simulink model "testPEConvSubmodule"  (R2023a)
settings: Solver=VariableStepAuto  StartTime=0.0  StopTime=simu.sim_time  MaxStep=simu.max_stepSize  RelTol=1e-3
values from neighbouring files (symbols this model uses):
  dev = peDevClass("default_mosfet")    [peModelingTest.m]
  i_rms = 25    [peModelingTest.m]
  ma = 0.98    [peModelingTest.m]
libraries: fl_lib x17, nesl_utility x5, simulink x1
settings Model: Creator=smbar  LastModifiedBy=bartonsa
settings DataIOCC: ReturnWorkspaceOutputs=off

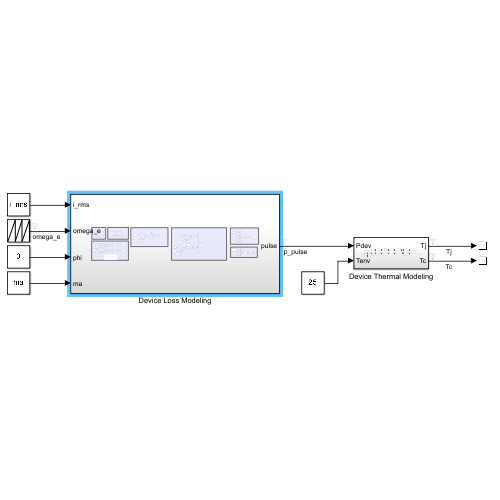
[thumbnail: Simulink's stored preview of the top-level diagram]
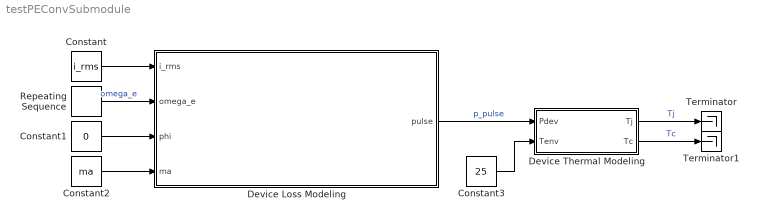
== system testPEConvSubmodule ==
  Constant : Constant  Value=i_rms
  Constant1 : Constant  Value=0
  Constant2 : Constant  Value=ma
  Constant3 : Constant  Value=25
  Device Loss Modeling : Subsystem
  Device Thermal Modeling : Subsystem
  Repeating Sequence : simulink/Sources/Repeating Sequence  rep_seq_t=time_vec  rep_seq_y=omega_e
  Terminator : Terminator
  Terminator1 : Terminator
  wires:
  Constant/1 -> Device Loss Modeling/1(i_rms)
  Repeating Sequence/1 -> Device Loss Modeling/2(omega_e)  "omega_e"
  Constant1/1 -> Device Loss Modeling/3(phi)
  Device Loss Modeling/1(pulse) -> Device Thermal Modeling/1(Pdev)  "p_pulse"
  Constant2/1 -> Device Loss Modeling/4(ma)
  Constant3/1 -> Device Thermal Modeling/2(Tenv)
  Device Thermal Modeling/2(Tc) -> Terminator1/1  "Tc"
  Device Thermal Modeling/1(Tj) -> Terminator/1  "Tj"

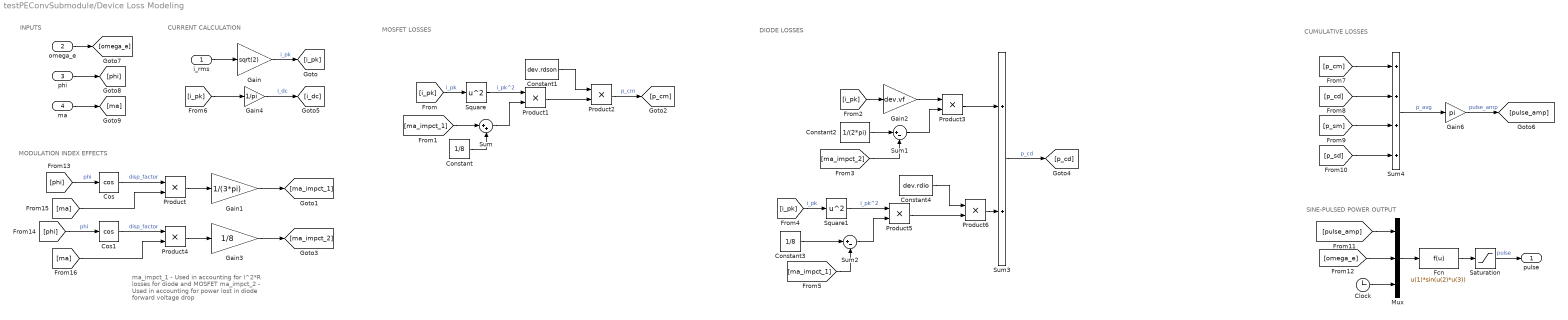
== system testPEConvSubmodule/Device Loss Modeling ==
  note: CUMULATIVE LOSSES
  note: DIODE LOSSES
  note: MOSFET LOSSES
  note: ma_impct_1 - Used in accounting for I^2*R losses for diode and MOSFET
      |
      | ma_impct_2 - Used in accounting for power lost in diode forward voltage drop
  note: MODULATION INDEX EFFECTS
  note: SINE-PULSED POWER OUTPUT
  note: CURRENT CALCULATION
  note: INPUTS
  i_rms : Inport
  omega_e : Inport  Port=2
  phi : Inport  Port=3
  ma : Inport  Port=4
  Clock : Clock
  Constant : Constant  Value=1/8
  Constant1 : Constant  Value=dev.rdson
  Constant2 : Constant  Value=1/(2*pi)
  Constant3 : Constant  Value=1/8
  Constant4 : Constant  Value=dev.rdio
  Cos : Trigonometry  Operator=cos
  Cos1 : Trigonometry  Operator=cos
  Fcn : Fcn  Expr=u(1)*sin(u(2)*u(3))
  Gain : Gain  Gain=sqrt(2)
  Gain1 : Gain  Gain=1/(3*pi)
  Gain2 : Gain  Gain=dev.vf
  Gain3 : Gain  Gain=1/8
  Gain4 : Gain  Gain=1/pi
  Gain6 : Gain  Gain=pi
  Mux : Mux  Inputs=3
  Product{,1..6} (7 alike) : Product
  Saturation : Saturate  UpperLimit=inf  LowerLimit=0
  Square : Math  Operator=square
  Square1 : Math  Operator=square
  Sum : Sum  Inputs=|++
  Sum1 : Sum  Inputs=|+-
  Sum2 : Sum  Inputs=|+-
  Sum3 : Sum
  Sum4 : Sum  Inputs=++++
  pulse : Outport
  wires:
  Product/1 -> Gain1/1
  Sum/1 -> Product1/2
  [pulse_amp] -> Mux/1
  [p_sm] -> Sum4/3
  Gain1/1 -> [ma_impct_1]
  [i_pk] -> Square/1  "i_pk"
  Gain6/1 -> [pulse_amp]  "pulse_amp"
  Sum3/1 -> [p_cd]  "p_cd"
  Product1/1 -> Product2/2
  Cos/1 -> Product/1  "disp_factor"
  Product5/1 -> Product6/2
  [i_pk] -> Square1/1  "i_pk"
  Gain/1 -> [i_pk]  "i_pk"
  Constant/1 -> Sum/2
  Square/1 -> Product1/1  "i_pk^2"
  [ma_impct_2] -> Sum1/2
  i_rms/1 -> Gain/1
  Sum1/1 -> Product3/2
  Product4/1 -> Gain3/1
  Product2/1 -> [p_cm]  "p_cm"
  [i_pk] -> Gain4/1
  Product3/1 -> Sum3/1
  [omega_e] -> Mux/2
  Constant1/1 -> Product2/1
  [i_pk] -> Gain2/1
  Constant4/1 -> Product6/1
  Gain4/1 -> [i_dc]  "i_dc"
  [phi] -> Cos1/1  "phi"
  [p_cd] -> Sum4/2
  [p_cm] -> Sum4/1
  Product6/1 -> Sum3/2
  [p_sd] -> Sum4/4
  [ma] -> Product4/2
  Sum4/1 -> Gain6/1  "p_avg"
  Fcn/1 -> Saturation/1
  [ma_impct_1] -> Sum/1
  Mux/1 -> Fcn/1
  [ma] -> Product/2
  Gain3/1 -> [ma_impct_2]
  Cos1/1 -> Product4/1  "disp_factor"
  Gain2/1 -> Product3/1
  Constant2/1 -> Sum1/1
  Square1/1 -> Product5/1  "i_pk^2"
  Clock/1 -> Mux/3
  Constant3/1 -> Sum2/1
  [ma_impct_1] -> Sum2/2
  Sum2/1 -> Product5/2
  [phi] -> Cos/1  "phi"
  omega_e/1 -> [omega_e]
  Saturation/1 -> pulse/1  "pulse"
  phi/1 -> [phi]
  ma/1 -> [ma]

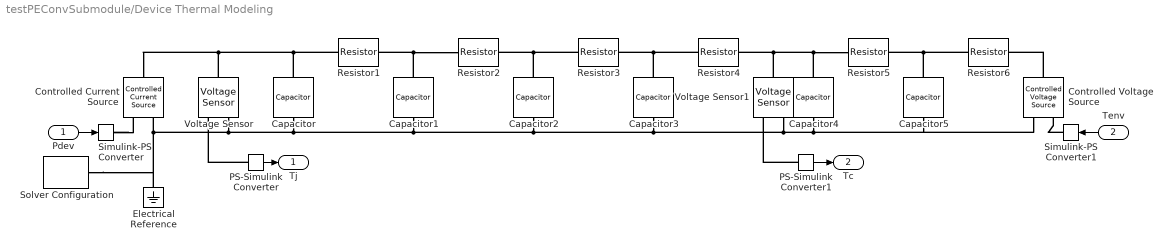
== system testPEConvSubmodule/Device Thermal Modeling ==
  Pdev : Inport
  Tenv : Inport  Port=2
  Capacitor : fl_lib/Electrical/Electrical Elements/Capacitor  c=dev.c(1) F  r=0 Ohm  g=0 1/Ohm  i_specify=off  i_priority=None  i=0 A  i_nominal_specify=off  i_nominal_unit=A  i_nominal_value=1  v_specify=off  v_priority=None  v=0 V  v_nominal_specify=off  v_nominal_unit=V  v_nominal_value=1  vc_specify=off  vc_priority=High  vc=0 V  vc_nominal_specify=off  vc_nominal_unit=V  vc_nominal_value=1
  Capacitor1 : fl_lib/Electrical/Electrical Elements/Capacitor  c=dev.c(2) F  r=0 Ohm  g=0 1/Ohm  i_specify=off  i_priority=None  i=0 A  i_nominal_specify=off  i_nominal_unit=A  i_nominal_value=1  v_specify=off  v_priority=None  v=0 V  v_nominal_specify=off  v_nominal_unit=V  v_nominal_value=1  vc_specify=off  vc_priority=High  vc=0 V  vc_nominal_specify=off  vc_nominal_unit=V  vc_nominal_value=1
  Capacitor2 : fl_lib/Electrical/Electrical Elements/Capacitor  c=dev.c(3) F  r=0 Ohm  g=0 1/Ohm  i_specify=off  i_priority=None  i=0 A  i_nominal_specify=off  i_nominal_unit=A  i_nominal_value=1  v_specify=off  v_priority=None  v=0 V  v_nominal_specify=off  v_nominal_unit=V  v_nominal_value=1  vc_specify=off  vc_priority=High  vc=0 V  vc_nominal_specify=off  vc_nominal_unit=V  vc_nominal_value=1
  Capacitor3 : fl_lib/Electrical/Electrical Elements/Capacitor  c=dev.c(4) F  r=0 Ohm  g=0 1/Ohm  i_specify=off  i_priority=None  i=0 A  i_nominal_specify=off  i_nominal_unit=A  i_nominal_value=1  v_specify=off  v_priority=None  v=0 V  v_nominal_specify=off  v_nominal_unit=V  v_nominal_value=1  vc_specify=off  vc_priority=High  vc=0 V  vc_nominal_specify=off  vc_nominal_unit=V  vc_nominal_value=1
  Capacitor4 : fl_lib/Electrical/Electrical Elements/Capacitor  c=dev.c(5) F  r=0 Ohm  g=0 1/Ohm  i_specify=off  i_priority=None  i=0 A  i_nominal_specify=off  i_nominal_unit=A  i_nominal_value=1  v_specify=off  v_priority=None  v=0 V  v_nominal_specify=off  v_nominal_unit=V  v_nominal_value=1  vc_specify=off  vc_priority=High  vc=0 V  vc_nominal_specify=off  vc_nominal_unit=V  vc_nominal_value=1
  Capacitor5 : fl_lib/Electrical/Electrical Elements/Capacitor  c=dev.c(6) F  r=0 Ohm  g=0 1/Ohm  i_specify=off  i_priority=None  i=0 A  i_nominal_specify=off  i_nominal_unit=A  i_nominal_value=1  v_specify=off  v_priority=None  v=0 V  v_nominal_specify=off  v_nominal_unit=V  v_nominal_value=1  vc_specify=off  vc_priority=High  vc=0 V  vc_nominal_specify=off  vc_nominal_unit=V  vc_nominal_value=1
  Controlled Current Source : fl_lib/Electrical/Electrical Sources/Controlled Current Source
  Controlled Voltage Source : fl_lib/Electrical/Electrical Sources/Controlled Voltage Source
  Electrical Reference : fl_lib/Electrical/Electrical Elements/Electrical Reference
  PS-Simulink Converter : nesl_utility/PS-Simulink Converter  PhysicalDomain=network_engine_domain  SubClassName=ps_output  LeftPortType=input  RightPortType=output  PseudoPeriodic=off  Frequencies=[]  VectorFormat=inherit  Unit=inherit  AffineConversion=off
  PS-Simulink Converter1 : nesl_utility/PS-Simulink Converter  PhysicalDomain=network_engine_domain  SubClassName=ps_output  LeftPortType=input  RightPortType=output  PseudoPeriodic=off  Frequencies=[]  VectorFormat=inherit  Unit=inherit  AffineConversion=off
  Resistor1 : fl_lib/Electrical/Electrical Elements/Resistor  R=dev.theta(1) Ohm  i_specify=off  i_priority=None  i=0 A  i_nominal_specify=off  i_nominal_unit=A  i_nominal_value=1  v_specify=off  v_priority=None  v=0 V  v_nominal_specify=off  v_nominal_unit=V  v_nominal_value=1
  Resistor2 : fl_lib/Electrical/Electrical Elements/Resistor  R=dev.theta(2) Ohm  i_specify=off  i_priority=None  i=0 A  i_nominal_specify=off  i_nominal_unit=A  i_nominal_value=1  v_specify=off  v_priority=None  v=0 V  v_nominal_specify=off  v_nominal_unit=V  v_nominal_value=1
  Resistor3 : fl_lib/Electrical/Electrical Elements/Resistor  R=dev.theta(3) Ohm  i_specify=off  i_priority=None  i=0 A  i_nominal_specify=off  i_nominal_unit=A  i_nominal_value=1  v_specify=off  v_priority=None  v=0 V  v_nominal_specify=off  v_nominal_unit=V  v_nominal_value=1
  Resistor4 : fl_lib/Electrical/Electrical Elements/Resistor  R=dev.theta(4) Ohm  i_specify=off  i_priority=None  i=0 A  i_nominal_specify=off  i_nominal_unit=A  i_nominal_value=1  v_specify=off  v_priority=None  v=0 V  v_nominal_specify=off  v_nominal_unit=V  v_nominal_value=1
  Resistor5 : fl_lib/Electrical/Electrical Elements/Resistor  R=dev.theta(5) Ohm  i_specify=off  i_priority=None  i=0 A  i_nominal_specify=off  i_nominal_unit=A  i_nominal_value=1  v_specify=off  v_priority=None  v=0 V  v_nominal_specify=off  v_nominal_unit=V  v_nominal_value=1
  Resistor6 : fl_lib/Electrical/Electrical Elements/Resistor  R=dev.theta(6) Ohm  i_specify=off  i_priority=None  i=0 A  i_nominal_specify=off  i_nominal_unit=A  i_nominal_value=1  v_specify=off  v_priority=None  v=0 V  v_nominal_specify=off  v_nominal_unit=V  v_nominal_value=1
  Simulink-PS Converter : nesl_utility/Simulink-PS Converter  PhysicalDomain=network_engine_domain  SubClassName=ps_input  LeftPortType=input  RightPortType=output  PseudoPeriodic=off  Frequencies=[]  NoiseDistribution=none  NoiseParameters=[]  Unit=1  AffineConversion=off  FilteringAndDerivatives=provide  SimscapeFilterOrder=1  InputFilterTimeConstant=0.001  UdotUserProvided=0
  Simulink-PS Converter1 : nesl_utility/Simulink-PS Converter  PhysicalDomain=network_engine_domain  SubClassName=ps_input  LeftPortType=input  RightPortType=output  PseudoPeriodic=off  Frequencies=[]  NoiseDistribution=none  NoiseParameters=[]  Unit=1  AffineConversion=off  FilteringAndDerivatives=provide  SimscapeFilterOrder=1  InputFilterTimeConstant=0.001  UdotUserProvided=0
  Solver Configuration : nesl_utility/Solver Configuration  PhysicalDomain=network_engine_domain  SubClassName=solver  LeftPortType=input  RightPortType=generic  Tones=[]  Harmonics=[]  SimulateNoise=off  Profile=off  UseLocalSampling=off  EnableSwitchedLinearOptims=on  FrequencyDomain=off  UseCCode=off  RelTol=0.001  AbsTol=0.001  MinStep=1e-09  ToWorkspace=off  RevertToSquareIcSolve=off  NumHomotopyIterations=100  PhasorMode=off  PhasorModeNumHarmonics=1  ConsistencySolver=NEWTON_XTOL_AFTER_FTOL  IndexReductionMethod=DerivativeReplacement  DoDC=off  ResidualTolerance=1e-09  ConsistencyTolSource=GLOBAL  ConsistencyAbsTol=0.001  ConsistencyRelTol=0.001  ConsistencyTolFactor=0.001  UseLocalSolver=off  LocalSolverChoice=NE_BACKWARD_EULER_ADVANCER  ResolveIndetEquations=on  FunctionEvalNumThread=1  LocalSolverSampleTime=0.001  DoFixedCost=off  MaxNonlinIter=3  MaxModeIter=2  ComputeImpulses=off  ImpulseIterations=2  LinearAlgebra=auto  LinearAlgebraNumThread=0  EquationFormulation=NE_TIME_EF  DelaysMemoryBudget=1024  AutomaticFiltering=on  FilteringTimeConstant=0.001  PartitionStorageMethod=AS_NEEDED  PartitionMemoryBudget=1024  PartitionMethod=ROBUST
  Voltage Sensor : fl_lib/Electrical/Electrical Sensors/Voltage Sensor
  Voltage Sensor1 : fl_lib/Electrical/Electrical Sensors/Voltage Sensor
  Tj : Outport
  Tc : Outport  Port=2
  wires:
  Pdev/1 -> Simulink-PS Converter/1
  Tenv/1 -> Simulink-PS Converter1/1
  PS-Simulink Converter/1 -> Tj/1
  PS-Simulink Converter1/1 -> Tc/1
  connections:
  Simulink-PS Converter/RConn1 -- Controlled Current Source/RConn1
  Capacitor/LConn1 -- Voltage Sensor/LConn1 -- Controlled Current Source/LConn1 -- Resistor1/LConn1
  Capacitor3/RConn1 -- Voltage Sensor1/RConn2 -- Controlled Voltage Source/RConn2 -- Capacitor5/RConn1 -- Capacitor4/RConn1 -- Voltage Sensor/RConn2 -- Solver Configuration/RConn1 -- Electrical Reference/LConn1 -- Controlled Current Source/RConn2 -- Capacitor/RConn1 -- Capacitor1/RConn1 -- Capacitor2/RConn1
  Capacitor1/LConn1 -- Resistor1/RConn1 -- Resistor2/LConn1
  Capacitor2/LConn1 -- Resistor2/RConn1 -- Resistor3/LConn1
  Capacitor4/LConn1 -- Resistor5/LConn1 -- Voltage Sensor1/LConn1 -- Resistor4/RConn1
  Capacitor3/LConn1 -- Resistor3/RConn1 -- Resistor4/LConn1
  Capacitor5/LConn1 -- Resistor5/RConn1 -- Resistor6/LConn1
  Controlled Voltage Source/LConn1 -- Resistor6/RConn1
  Simulink-PS Converter1/RConn1 -- Controlled Voltage Source/RConn1
  PS-Simulink Converter/LConn1 -- Voltage Sensor/RConn1
  PS-Simulink Converter1/LConn1 -- Voltage Sensor1/RConn1
